simulink model "modeloMike"  (R2020a)
settings: Solver=ode45  StartTime=0.0  StopTime=10  RelTol=1e-3  EnableMultiTasking=on
undefined symbols (not defined in the file): q1, q2, q3, r1, x1_0, x2_0, x3_0, x4_0
settings Model: Creator=Guillermo  LastModifiedBy=mique
settings DataIOCC: LimitDataPoints=on  SaveFormat=Array  SignalLoggingSaveFormat=ModelDataLogs  ReturnWorkspaceOutputs=off
settings OptimizationCC: ExpressionDepthLimit=2147483647  InitFltsAndDblsToZero=on  LifeSpan=inf
settings DebuggingCC: SaveWithParameterizedLinksMsg=none  UnderspecifiedInitializationDetection=Classic  MergeDetectMultiDrivingBlocksExec=none  SignalResolutionControl=TryResolveAllWithWarning  SolverPrmCheckMsg=warning  MultiTaskDSMMsg=warning  MultiTaskCondExecSysMsg=none  FcnCallInpInsideContextMsg=warning  StateNameClashWarn=warning  SFUnexpectedBacktrackingDiag=warning  SFNoUnconditionalDefaultTransitionDiag=warning  SFExecutionAtInitializationDiag=none  ArithmeticOperatorsInVariantConditions=warning
settings HardwareCC: ProdBitPerPointer=32  ProdBitPerSizeT=32  ProdBitPerPtrDiffT=32  ProdLargestAtomicFloat=None  ProdIntDivRoundTo=Undefined  ProdEndianess=Unspecified  ProdWordSize=32  ProdHWDeviceType=32-bit Generic
settings ModelReferenceCC: PropagateSignalLabelsOutOfModel=off
settings SFSimCC: SimUseLocalCustomCode=off  CustomCodeUndefinedFunction=UseInterfaceOnly
settings RTWCC: RTWUseLocalCustomCode=off
settings CodeAppCC: StateflowObjectComments=on
settings GRTTargetCC: TargetFcnLib=ansi_tfl_tmw.mat  TargetLangStandard=C89/C90 (ANSI)  CombineOutputUpdateFcns=off  GRTInterface=on
settings ConfigComp: CovMetricSettings=dw  CovHtmlReporting=on  CovSaveCumulativeToWorkspaceVar=on  CovSaveSingleToWorkspaceVar=on  CovExternalEMLEnable=off

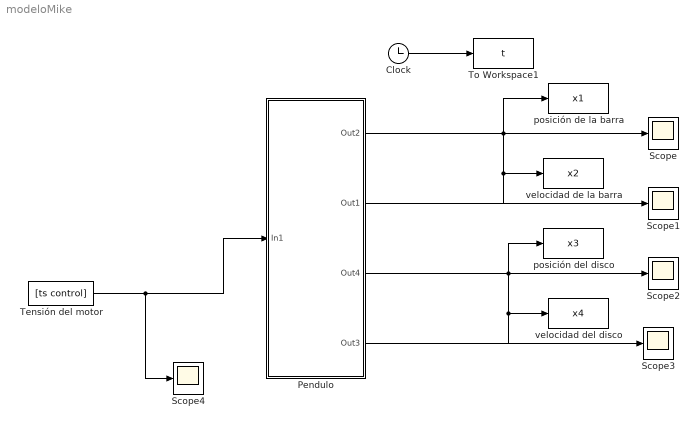
== system modeloMike ==
  Clock : Clock
  Pendulo : Subsystem
  Scope{,1..4} (5 alike) : Scope
  Tensión del motor : FromWorkspace  VariableName=[ts control]  SampleTime=0.01  ZeroCross=off
  To Workspace1 : ToWorkspace  VariableName=t  SampleTime=-1
  posición de la barra : ToWorkspace  VariableName=x1  SampleTime=-1
  posición del disco : ToWorkspace  VariableName=x3  SampleTime=-1
  velocidad de la barra : ToWorkspace  VariableName=x2  SampleTime=-1
  velocidad del disco : ToWorkspace  VariableName=x4  SampleTime=-1
  wires:
  Clock/1 -> To Workspace1/1
  Pendulo/2(Out1) -> Scope/1, posición de la barra/1
  Pendulo/1(Out2) -> Scope1/1, velocidad de la barra/1
  Pendulo/4(Out3) -> posición del disco/1, Scope2/1
  Pendulo/3(Out4) -> Scope3/1, velocidad del disco/1
  Tensión del motor/1 -> Scope4/1, Pendulo/1(In1)

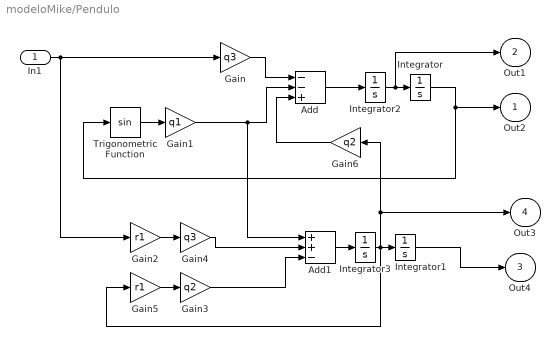
== system modeloMike/Pendulo ==
  In1 : Inport  PortDimensions=1
  Add : Sum  Inputs=--+
  Add1 : Sum  Inputs=++-
  Gain : Gain  Gain=q3
  Gain1 : Gain  Gain=q1
  Gain2 : Gain  Gain=r1
  Gain3 : Gain  Gain=q2
  Gain4 : Gain  Gain=q3
  Gain5 : Gain  Gain=r1
  Gain6 : Gain  Gain=q2
  Integrator : Integrator  InitialCondition=x1_0
  Integrator1 : Integrator  InitialCondition=x3_0
  Integrator2 : Integrator  InitialCondition=x2_0
  Integrator3 : Integrator  InitialCondition=x4_0
  Trigonometric Function : Trigonometry
  Out2 : Outport
  Out1 : Outport  Port=2
  Out4 : Outport  Port=3
  Out3 : Outport  Port=4
  wires:
  Trigonometric Function/1 -> Gain1/1
  Gain1/1 -> Add1/1, Add/2
  Add/1 -> Integrator2/1
  Gain/1 -> Add/1
  In1/1 -> Gain/1, Gain2/1
  Gain5/1 -> Gain3/1
  Gain3/1 -> Add1/3
  Add1/1 -> Integrator3/1
  Gain2/1 -> Gain4/1
  Integrator/1 -> Trigonometric Function/1, Out2/1
  Integrator2/1 -> Integrator/1, Out1/1
  Integrator3/1 -> Gain5/1, Integrator1/1, Gain6/1, Out3/1
  Gain4/1 -> Add1/2
  Gain6/1 -> Add/3
  Integrator1/1 -> Out4/1
